simulink model "temperatur"  (R2025a)
settings: Solver=VariableStepAuto  StartTime=0.0  StopTime=20000  RelTol=1e-3
values from neighbouring files (symbols this model uses):
  c = 1000    [romtemperatur_init.m]
  rho = 1.225    [romtemperatur_init.m]
  U = 0.5    [romtemperatur_init.m]
  V = 30    [romtemperatur_init.m]
settings Model: Creator=emcoates  LastModifiedBy=user

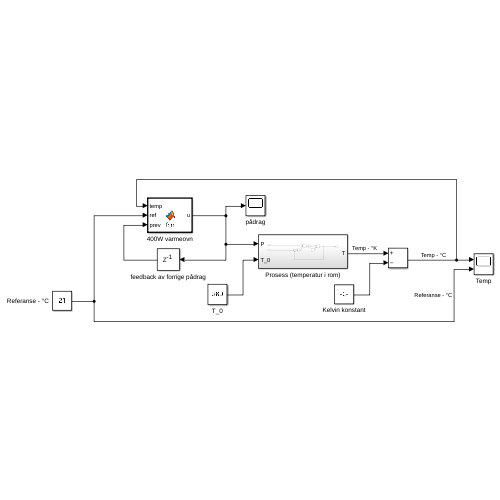
[thumbnail: Simulink's stored preview of the top-level diagram]
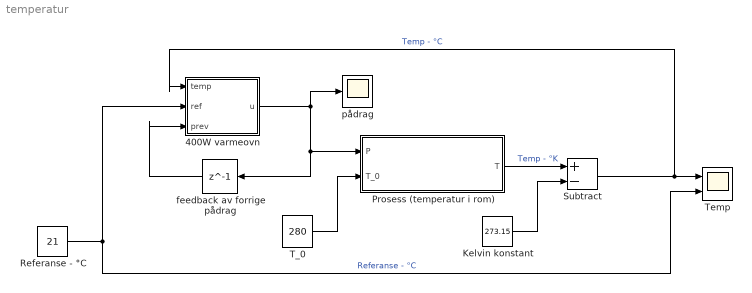
== system temperatur ==
  400W varmeovn : MATLAB Function  TreatAsAtomicUnit=on
  Kelvin konstant : Constant  Value=273.15
  Prosess (temperatur i rom) : Subsystem
  Referanse - °C : Constant  Value=21
  Subtract : Sum  Inputs=+-
  T_0 : Constant  Value=280
  Temp : Scope  NumInputPorts=2
      settings: ActiveDisplayYMinimum=8.35348041990148  ActiveDisplayYMaximum=24.81867622088668
  feedback av forrige pådrag : Delay  DelayLength=1
  pådrag : Scope
      settings: ActiveDisplayYMinimum=-49.999999999999986  ActiveDisplayYMaximum=450
  wires:
  T_0/1 -> Prosess (temperatur i rom)/2(T_0)
  Prosess (temperatur i rom)/1(T) -> Subtract/1  "Temp - °K"
  400W varmeovn/1(u) -> feedback av forrige pådrag/1, Prosess (temperatur i rom)/1(P), pådrag/1
  Subtract/1 -> Temp/1, 400W varmeovn/1(temp)  "Temp - °C"
  Kelvin konstant/1 -> Subtract/2
  Referanse - °C/1 -> Temp/2, 400W varmeovn/2(ref)  "Referanse - °C"
  feedback av forrige pådrag/1 -> 400W varmeovn/3(prev)

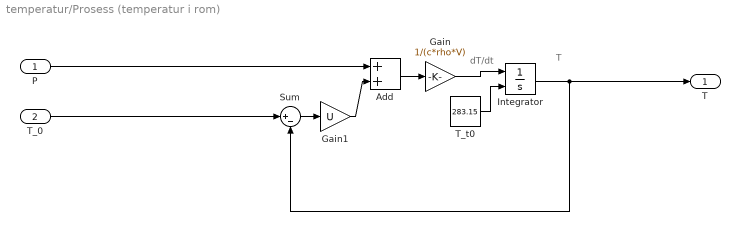
== system temperatur/Prosess (temperatur i rom) ==
  note: T
  note: dT/dt
  P : Inport
  T_0 : Inport  Port=2
  Add : Sum
  Gain : Gain  Gain=1/(c*rho*V)
  Gain1 : Gain  Gain=U
  Integrator : Integrator  InitialConditionSource=external
  Sum : Sum  Inputs=|+-
  T_t0 : Constant  Value=283.15
  T : Outport
  wires:
  Gain1/1 -> Add/2
  Integrator/1 -> T/1, Sum/2
  Gain/1 -> Integrator/1
  T_0/1 -> Sum/1
  Add/1 -> Gain/1
  T_t0/1 -> Integrator/2
  Sum/1 -> Gain1/1
  P/1 -> Add/1

== matlab function temperatur/400W varmeovn ==
  data: temp input; u output; ref input; prev input
function u = fcn(temp, ref, prev)

on = 400; % Watt
off = 0;

hysterese = 0.5; % °C

if temp <= ref+hysterese && temp >= ref-hysterese
    u = prev;
elseif temp < ref
    u = on;
else 
    u = off;
end
